simulink model "modelos"  (R2020b)
settings: Solver=VariableStepAuto  StartTime=0.0  StopTime=300  RelTol=1e-3
settings Model: Creator=ian  LastModifiedBy=ian

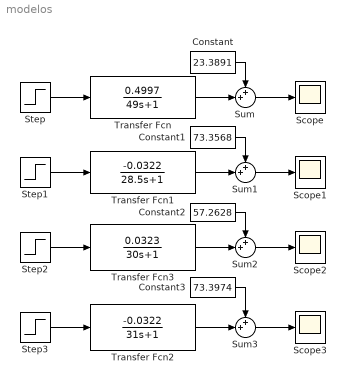
== system modelos ==
  Constant : Constant  Value=23.3891
  Constant1 : Constant  Value=73.3568
  Constant2 : Constant  Value=57.2628
  Constant3 : Constant  Value=73.3974
  Scope{,1..3} (4 alike) : Scope
  Step : Step  After=100  SampleTime=0
  Step1 : Step  After=500  SampleTime=0
  Step2 : Step  After=500  SampleTime=0
  Step3 : Step  After=1000  SampleTime=0
  Sum{,1..3} (4 alike) : Sum  Inputs=++|
  Transfer Fcn : TransferFcn  Numerator=[0.4997]  Denominator=[49 1]
  Transfer Fcn1 : TransferFcn  Numerator=[-0.0322]  Denominator=[28.5 1]
  Transfer Fcn2 : TransferFcn  Numerator=[-0.0322]  Denominator=[31 1]
  Transfer Fcn3 : TransferFcn  Numerator=[0.0323]  Denominator=[30 1]
  wires:
  Step/1 -> Transfer Fcn/1
  Step1/1 -> Transfer Fcn1/1
  Step2/1 -> Transfer Fcn3/1
  Step3/1 -> Transfer Fcn2/1
  Transfer Fcn/1 -> Sum/2
  Constant/1 -> Sum/1
  Sum/1 -> Scope/1
  Transfer Fcn1/1 -> Sum1/2
  Sum1/1 -> Scope1/1
  Constant1/1 -> Sum1/1
  Constant2/1 -> Sum2/1
  Constant3/1 -> Sum3/1
  Transfer Fcn3/1 -> Sum2/2
  Sum2/1 -> Scope2/1
  Sum3/1 -> Scope3/1
  Transfer Fcn2/1 -> Sum3/2
